simulink model "hoop_pose_2022a"  (R2022a)
settings: Solver=VariableStepAuto  StartTime=0.0  StopTime=10.0  RelTol=1e-3
libraries: robotlib x5
settings Model: Creator=cftemp3  LastModifiedBy=enriq
settings DebuggingCC: UnconnectedInputMsg=warning  UnconnectedOutputMsg=warning  UnconnectedLineMsg=warning
settings RTWCC: DLArmComputeVersion=19.05

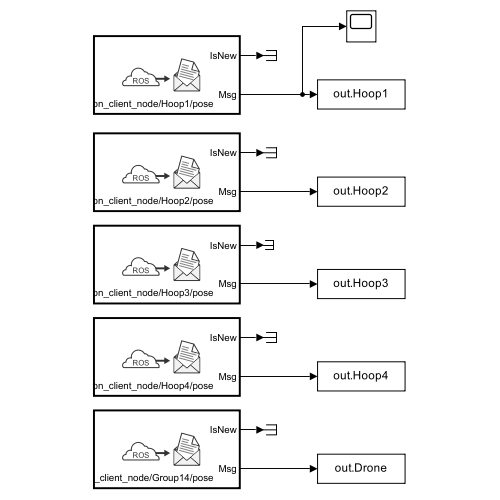
[thumbnail: Simulink's stored preview of the top-level diagram]
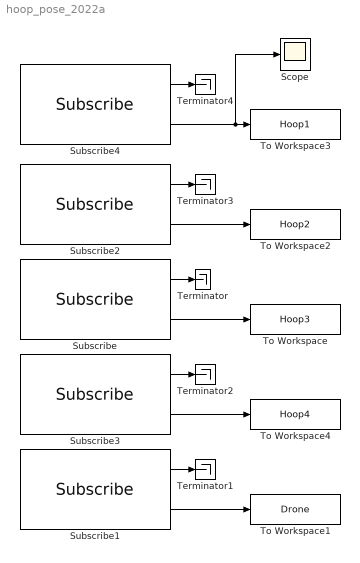
== system hoop_pose_2022a ==
  Scope : Scope
  Subscribe : robotlib/Subscribe  topicSource=Select from ROS network  topic=/vrpn_client_node/Hoop3/pose  messageType=geometry_msgs/PoseStamped  SampleTime=-1  legacyBusStruct=off  messageQueueLength=1
  Subscribe1 : robotlib/Subscribe  topicSource=Select from ROS network  topic=/vrpn_client_node/Group14/pose  messageType=geometry_msgs/PoseStamped  SampleTime=-1  legacyBusStruct=off  messageQueueLength=1
  Subscribe2 : robotlib/Subscribe  topicSource=Select from ROS network  topic=/vrpn_client_node/Hoop2/pose  messageType=geometry_msgs/PoseStamped  SampleTime=-1  legacyBusStruct=off  messageQueueLength=1
  Subscribe3 : robotlib/Subscribe  topicSource=Select from ROS network  topic=/vrpn_client_node/Hoop4/pose  messageType=geometry_msgs/PoseStamped  SampleTime=-1  legacyBusStruct=off  messageQueueLength=1
  Subscribe4 : robotlib/Subscribe  topicSource=Select from ROS network  topic=/vrpn_client_node/Hoop1/pose  messageType=geometry_msgs/PoseStamped  SampleTime=-1  legacyBusStruct=off  messageQueueLength=1
  Terminator{,1..4} (5 alike) : Terminator
  To Workspace : ToWorkspace  VariableName=Hoop3  SaveFormat=Timeseries  SampleTime=-1
  To Workspace1 : ToWorkspace  VariableName=Drone  SaveFormat=Timeseries  SampleTime=-1
  To Workspace2 : ToWorkspace  VariableName=Hoop2  SaveFormat=Timeseries  SampleTime=-1
  To Workspace3 : ToWorkspace  VariableName=Hoop1  SaveFormat=Timeseries  SampleTime=-1
  To Workspace4 : ToWorkspace  VariableName=Hoop4  SaveFormat=Timeseries  SampleTime=-1
  wires:
  Subscribe4/2 -> Scope/1, To Workspace3/1
  Subscribe2/2 -> To Workspace2/1
  Subscribe/2 -> To Workspace/1
  Subscribe3/2 -> To Workspace4/1
  Subscribe1/2 -> To Workspace1/1
  Subscribe1/1 -> Terminator1/1
  Subscribe3/1 -> Terminator2/1
  Subscribe/1 -> Terminator/1
  Subscribe2/1 -> Terminator3/1
  Subscribe4/1 -> Terminator4/1
